simulink library "csu_dmo_dtu_message_output_lib"  (R2015b)
settings: Solver=ode45  SolverMode=SingleTasking  StartTime=0.0  StopTime=10.0  RelTol=1e-3
libraries: util_common_lib x7, util_info_lib x1
settings Model: Creator=hcannon  LastModifiedBy=jimkaidy
settings DataIOCC: SaveFormat=Array  SignalLoggingSaveFormat=ModelDataLogs
settings OptimizationCC: BlockReduction=off  BooleanDataType=off  ExpressionDepthLimit=2147483647
settings DebuggingCC: SaveWithParameterizedLinksMsg=none  UnderspecifiedInitializationDetection=Classic  MergeDetectMultiDrivingBlocksExec=none  SignalResolutionControl=TryResolveAllWithWarning  FcnCallInpInsideContextMsg=EnableAllAsWarning  StateNameClashWarn=warning  StrictBusMsg=Warning
settings HardwareCC: ProdBitPerPointer=32  ProdLargestAtomicFloat=None  ProdIntDivRoundTo=Undefined  ProdEndianess=Unspecified  ProdWordSize=32  ProdHWDeviceType=32-bit Generic  TargetUnknown=on
settings GRTTargetCC: GeneratePreprocessorConditionals=Disable all
settings ConfigComp: CovModelRefEnable=Off  CovSFcnEnable=off

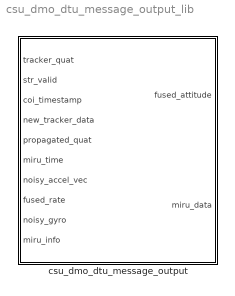
== system csu_dmo_dtu_message_output_lib ==
  csu_dmo_dtu_message_output : Subsystem

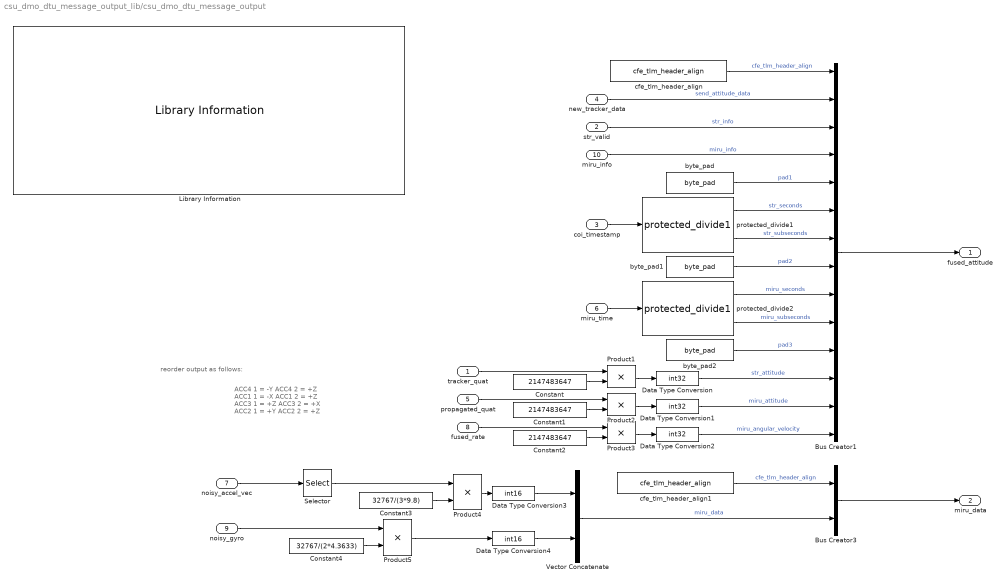
== system csu_dmo_dtu_message_output_lib/csu_dmo_dtu_message_output ==
  note: reorder output as follows:
  note: ACC4 1 = -Y
      | ACC4 2 = +Z
      | ACC1 1 = -X
      | ACC1 2 = +Z
      | ACC3 1 = +Z
      | ACC3 2 = +X
      | ACC2 1 = +Y
      | ACC2 2 = +Z
  tracker_quat : Inport
  str_valid : Inport  Port=2
  coi_timestamp : Inport  Port=3
  new_tracker_data : Inport  Port=4
  propagated_quat : Inport  Port=5
  miru_time : Inport  Port=6
  noisy_accel_vec : Inport  Port=7
  fused_rate : Inport  Port=8
  noisy_gyro : Inport  Port=9
  miru_info : Inport  Port=10
  Bus Creator1 : BusCreator  Inputs=14  OutDataTypeStr=Bus: fused_attitude_msg  NonVirtualBus=on
  Bus Creator3 : BusCreator  Inputs=2  OutDataTypeStr=Bus: miru_data_msg  NonVirtualBus=on
  Constant : Constant  Value=2147483647  OutDataTypeStr=double
  Constant1 : Constant  Value=2147483647  OutDataTypeStr=double
  Constant2 : Constant  Value=2147483647  OutDataTypeStr=double
  Constant3 : Constant  Value=32767/(3*9.8)  OutDataTypeStr=double
  Constant4 : Constant  Value=32767/(2*4.3633)  OutDataTypeStr=double
  Data Type Conversion : DataTypeConversion  OutDataTypeStr=int32
  Data Type Conversion1 : DataTypeConversion  OutDataTypeStr=int32
  Data Type Conversion2 : DataTypeConversion  OutDataTypeStr=int32
  Data Type Conversion3 : DataTypeConversion  OutDataTypeStr=int16
  Data Type Conversion4 : DataTypeConversion  OutDataTypeStr=int16
  Library Information : util_info_lib/Library Information  owner='escrane'
  Product{1..5} (5 alike) : Product  RndMeth=Zero
  Selector : Selector  InputPortWidth=8  IndexOptions=Index vector (dialog)  Indices=[7 8 1 2 5 6 3 4]  OutputSizes=1
  Vector Concatenate : Concatenate
  byte_pad : util_common_lib/byte_pad  n_bytes=1
  byte_pad1 : util_common_lib/byte_pad  n_bytes=2
  byte_pad2 : util_common_lib/byte_pad  n_bytes=2
  cfe_tlm_header_align : util_common_lib/cfe_tlm_header_align
  cfe_tlm_header_align1 : util_common_lib/cfe_tlm_header_align
  protected_divide1 : util_common_lib/protected_divide1  SystemSampleTime=-1
  protected_divide2 : util_common_lib/protected_divide1  SystemSampleTime=-1
  fused_attitude : Outport
  miru_data : Outport  Port=2
  wires:
  Data Type Conversion4/1 -> Vector Concatenate/2
  Product5/1 -> Data Type Conversion4/1
  Constant4/1 -> Product5/2
  noisy_gyro/1 -> Product5/1
  Data Type Conversion3/1 -> Vector Concatenate/1
  Product4/1 -> Data Type Conversion3/1
  Constant3/1 -> Product4/2
  Selector/1 -> Product4/1
  Data Type Conversion2/1 -> Bus Creator1/14  "miru_angular_velocity"
  Product3/1 -> Data Type Conversion2/1
  Constant2/1 -> Product3/2
  Data Type Conversion1/1 -> Bus Creator1/13  "miru_attitude"
  Product2/1 -> Data Type Conversion1/1
  Constant1/1 -> Product2/2
  propagated_quat/1 -> Product2/1
  Data Type Conversion/1 -> Bus Creator1/12  "str_attitude"
  Product1/1 -> Data Type Conversion/1
  Constant/1 -> Product1/2
  byte_pad2/1 -> Bus Creator1/11  "pad3"
  byte_pad1/1 -> Bus Creator1/8  "pad2"
  byte_pad/1 -> Bus Creator1/5  "pad1"
  noisy_accel_vec/1 -> Selector/1
  Bus Creator1/1 -> fused_attitude/1
  miru_info/1 -> Bus Creator1/4  "miru_info"
  fused_rate/1 -> Product3/1
  protected_divide1/1 -> Bus Creator1/6  "str_seconds"
  coi_timestamp/1 -> protected_divide1/1
  str_valid/1 -> Bus Creator1/3  "str_info"
  tracker_quat/1 -> Product1/1
  new_tracker_data/1 -> Bus Creator1/2  "send_attitude_data"
  cfe_tlm_header_align/1 -> Bus Creator1/1  "cfe_tlm_header_align"
  cfe_tlm_header_align1/1 -> Bus Creator3/1  "cfe_tlm_header_align"
  Vector Concatenate/1 -> Bus Creator3/2  "miru_data"
  Bus Creator3/1 -> miru_data/1
  protected_divide1/2 -> Bus Creator1/7  "str_subseconds"
  protected_divide2/1 -> Bus Creator1/9  "miru_seconds"
  protected_divide2/2 -> Bus Creator1/10  "miru_subseconds"
  miru_time/1 -> protected_divide2/1
